simulink model "pr643_PLL2_linear_model"  (R2018b)
settings: Solver=VariableStepAuto  StartTime=0.0  StopTime=1  RelTol=1e-3
values from neighbouring files (symbols this model uses):
  k1 = 0.1    [pr643_configure_PLL2_linear_model.m]    (also in test643.mat)
  k2 = (ko*kp*k1^2)/(4*d^2)    (= 0.01)    [pr643_configure_PLL2_linear_model.m]    (also in test643.mat)
  ko = 1    [pr643_configure_PLL2_linear_model.m]    (also in test643.mat)
  kp = 1    [pr643_configure_PLL2_linear_model.m]    (also in test643.mat)
libraries: simulink x1
settings Model: Creator=Григорий Фокин  LastModifiedBy=Григорий Фокин

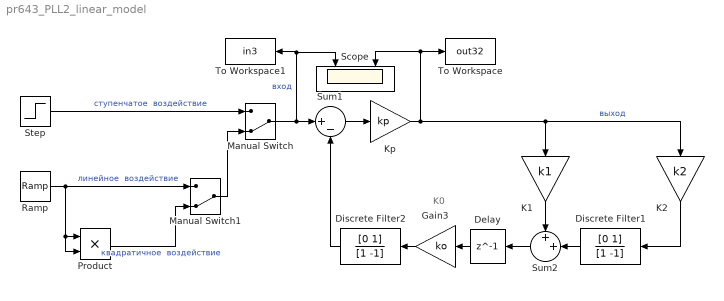
== system pr643_PLL2_linear_model ==
  note: K0
  Delay : Delay  DelayLength=1  InitialCondition=0
  Discrete Filter1 : DiscreteFilter  Numerator=[0 1]  Denominator=[1 -1]  SampleTime=1/1000
  Discrete Filter2 : DiscreteFilter  Numerator=[0 1]  Denominator=[1 -1]  SampleTime=1/1000
  Gain3 : Gain  Gain=ko
  K1 : Gain  Gain=k1
  K2 : Gain  Gain=k2
  Kp : Gain  Gain=kp
  Manual Switch : ManualSwitch  CurrentSetting=0
  Manual Switch1 : ManualSwitch  CurrentSetting=0
  Product : Product
  Ramp : simulink/Sources/Ramp  slope=2  start=0.2  InitialOutput=0
  Scope : Scope  NumInputPorts=2
  Step : Step  Time=0.2  SampleTime=1/1000
  Sum1 : Sum  Inputs=|+-
  Sum2 : Sum  Inputs=++|
  To Workspace : ToWorkspace  VariableName=out32  SaveFormat=Timeseries  SampleTime=-1
  To Workspace1 : ToWorkspace  VariableName=in3  SaveFormat=Timeseries  SampleTime=-1
  wires:
  Step/1 -> Manual Switch/1  "ступенчатое  воздействие"
  Ramp/1 -> Manual Switch1/1, Product/2, Product/1  "линейное  воздействие"
  Product/1 -> Manual Switch1/2  "квадратичное  воздействие"
  Manual Switch/1 -> Scope/1, To Workspace1/1, Sum1/1  "вход"
  K1/1 -> Sum2/1
  Discrete Filter1/1 -> Sum2/2
  K2/1 -> Discrete Filter1/1
  Sum2/1 -> Delay/1
  Delay/1 -> Gain3/1
  Gain3/1 -> Discrete Filter2/1
  Discrete Filter2/1 -> Sum1/2
  Sum1/1 -> Kp/1
  Kp/1 -> Scope/2, To Workspace/1, K2/1, K1/1  "выход"
  Manual Switch1/1 -> Manual Switch/2
